simulink model "aerosonde_dynamics_with_autopilot"  (R2021b)
settings: Solver=ode3  StartTime=0.0  StopTime=250  FixedStep=dt  RelTol=1e-6  EnableMultiTasking=on
InitFcn:
  | aerosonde_initialize
  | fault_configurations
  | init_sensor_model
StopFcn:
  | aerosende_grafik;
values from neighbouring files (symbols this model uses):
  aerosonde = AircraftSimData    [aerosonde_data.m]    (also in aerosonde_initialize.m = aerosonde_data)
  aoa_sensor_measurement_limit_rad = deg2rad(30)    [init_sensor_model.m]
  aoa_sensor_noise_power = 0.00030462    [init_sensor_model.m]
  bias_fault_active = TRUE    (= 1)    [fault_configurations.m]
  bias_fault_time = 150    [fault_configurations.m]
  bias_rad = deg2rad(3)    [fault_configurations.m]
  drift_fault_active = FALSE    (= 0)    [fault_configurations.m]
  drift_limit_rad = deg2rad(20)    [fault_configurations.m]
  drift_ratio_rad_s = deg2rad(0.2)    [fault_configurations.m]
  dt = 1/50    (= 0.02)    [aerosonde_initialize.m]
  F = [0 1 0 ... (first row only)    [aerosonde_initialize.m]
  flightconfig = flightconfig_data    [aerosonde_initialize.m]    (also in flightconfig_data.m = siminitialdetails)
  stuck_fault_active = FALSE    (= 0)    [fault_configurations.m]
  x_init = [510.0; -flightconfig.We_VL  ; 0.0]    [aerosonde_initialize.m]
undefined symbols (not defined in the file or in its folder): magnitude, MIL
libraries: simulink_extras x24, simulink x6, aerolibasang x3, aerolibwind2 x3, aerolibbdyn x2, aerolibadyn x1, aerolibtransform2 x1, shareddyn x1, aerolibobsolete x1, sharedutil x1, aerolibatmos2 x1
(part 2 of 2)

== system aerosonde_dynamics_with_autopilot/ UAV Dynamics/Total Moment ==
  note: Sum forces and moments
  note: Total moments at CG location
  Faero : Inport  PortDimensions=3
  Maero : Inport  Port=2  PortDimensions=3
  Fprop : Inport  Port=3  PortDimensions=3
  Mprop : Inport  Port=4  PortDimensions=3
  CGpos : Inport  Port=5  PortDimensions=3
  Moments about CG due to Propulsion Forces : aerolibbdyn/Moments about CG  due to Forces
      settings: SourceProductBaseCode=AE
  Sum1 : Sum  Inputs=+++  InputSameDT=on  SaturateOnIntegerOverflow=on  OutDataTypeStr=Inherit: Same as first input
  Total forces (excluding g) : Sum  InputSameDT=on  SaturateOnIntegerOverflow=on  OutDataTypeStr=Inherit: Same as first input
  r_prop : Constant  Value=aerosonde.rHub  OutDataTypeStr=double
  Fcg : Outport
  Mcg : Outport  Port=2
  wires:
  Maero/1 -> Sum1/2
  Moments about CG due to Propulsion Forces/1 -> Sum1/1
  Total forces (excluding g)/1 -> Fcg/1
  Faero/1 -> Total forces (excluding g)/1
  Fprop/1 -> Total forces (excluding g)/2, Moments about CG due to Propulsion Forces/1
  Mprop/1 -> Sum1/3
  Sum1/1 -> Mcg/1
  r_prop/1 -> Moments about CG due to Propulsion Forces/3
  CGpos/1 -> Moments about CG due to Propulsion Forces/2

== system aerosonde_dynamics_with_autopilot/AoA Sensor Model/Enabled Subsystem ==
  alpha_fault_free : Inport
  Enable : EnablePort
  Add : Sum
  Clock : Clock
  Constant : Constant  Value=bias_fault_time
  Constant1 : Constant  Value=bias_rad
  GreaterThan : RelationalOperator  Operator=>  OutDataTypeStr=boolean  RndMeth=Simplest
  Product : Product
  Transfer Fcn : TransferFcn  Denominator=[0.1 1]
  alpha_biased_rad : Outport
  wires:
  Clock/1 -> GreaterThan/1
  Constant/1 -> GreaterThan/2
  GreaterThan/1 -> Product/1
  Constant1/1 -> Product/2
  Product/1 -> Transfer Fcn/1
  alpha_fault_free/1 -> Add/1
  Transfer Fcn/1 -> Add/2
  Add/1 -> alpha_biased_rad/1

== system aerosonde_dynamics_with_autopilot/AoA Sensor Model/Enabled Subsystem1 ==
  alpha_fault_free : Inport
  Enable : EnablePort
  Add : Sum
  Clock : Clock
  Constant : Constant  Value=bias_fault_time
  Constant1 : Constant  Value=drift_ratio_rad_s
  GreaterThan : RelationalOperator  Operator=>  OutDataTypeStr=boolean  RndMeth=Simplest
  Integrator : Integrator  LimitOutput=on  UpperSaturationLimit=drift_limit_rad  LowerSaturationLimit=-drift_limit_rad
  Product : Product
  alpha_drifted_rad : Outport
  wires:
  Add/1 -> alpha_drifted_rad/1
  Integrator/1 -> Add/2
  alpha_fault_free/1 -> Add/1
  Product/1 -> Integrator/1
  Constant1/1 -> Product/2
  GreaterThan/1 -> Product/1
  Constant/1 -> GreaterThan/2
  Clock/1 -> GreaterThan/1

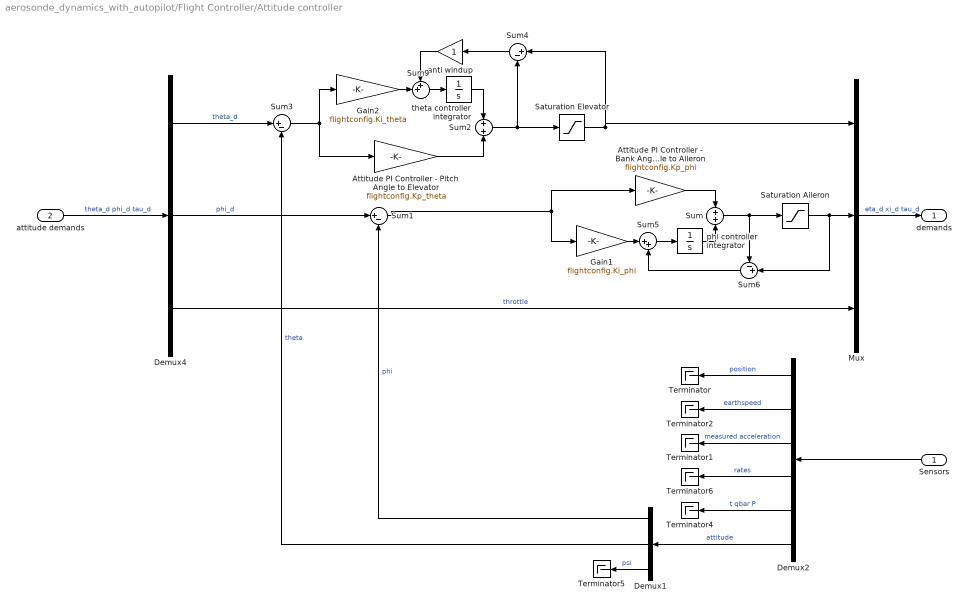
== system aerosonde_dynamics_with_autopilot/Flight Controller/Attitude controller ==
  Sensors : Inport
  attitude demands : Inport  Port=2
  Attitude PI Controller - Bank Angle to Aileron : Gain  Gain=flightconfig.Kp_phi
  Attitude PI Controller - Pitch Angle to Elevator : Gain  Gain=flightconfig.Kp_theta
  Demux1 : Demux  Outputs=3
      settings: DisplayOption=none
  Demux2 : Demux  Outputs=[3 3 3 3 3 3]
  Demux4 : Demux  Outputs=3
      settings: DisplayOption=none
  Gain1 : Gain  Gain=flightconfig.Ki_phi
  Gain2 : Gain  Gain=flightconfig.Ki_theta
  Mux : Mux  Inputs=3
  Saturation Aileron : Saturate  UpperLimit=20*pi/180  LowerLimit=-20*pi/180  ZeroCross=off
  Saturation Elevator : Saturate  UpperLimit=20*pi/180  LowerLimit=-20*pi/180  ZeroCross=off
  Sum : Sum  Inputs=+|+
  Sum1 : Sum  Inputs=|+-
  Sum2 : Sum  Inputs=+|+
  Sum3 : Sum  Inputs=|+-
  Sum4 : Sum  Inputs=|+-
  Sum5 : Sum  Inputs=|++
  Sum6 : Sum  Inputs=-+|
  Sum9 : Sum  Inputs=++|
  Terminator{,1..2,4..6} (6 alike) : Terminator
  anti windup : Gain
  phi controller integrator : Integrator  InitialCondition=flightconfig.xi_trim
  theta controller integrator : Integrator  InitialCondition=flightconfig.eta_trim + flightconfig.Ktheta_eta*flightconfig.theta_trim + flightconfig.Kq_eta*flightconfig.q_trim
  demands : Outport
  wires:
  Sum1/1 -> Attitude PI Controller - Bank Angle to Aileron/1, Gain1/1
  Demux4/2 -> Sum1/1  "phi_d"
  Sum3/1 -> Gain2/1, Attitude PI Controller - Pitch Angle to Elevator/1
  theta controller integrator/1 -> Sum2/1
  Attitude PI Controller - Pitch Angle to Elevator/1 -> Sum2/2
  Gain2/1 -> Sum9/2
  Sum9/1 -> theta controller integrator/1
  Sum2/1 -> Saturation Elevator/1, Sum4/2
  Saturation Elevator/1 -> Sum4/1, Mux/1
  Sum4/1 -> anti windup/1
  anti windup/1 -> Sum9/1
  phi controller integrator/1 -> Sum/2
  Sum/1 -> Saturation Aileron/1, Sum6/1
  Demux4/3 -> Mux/3  "throttle"
  attitude demands/1 -> Demux4/1  "theta_d phi_d tau_d"
  Mux/1 -> demands/1  "eta_d xi_d tau_d"
  Demux4/1 -> Sum3/1  "theta_d"
  Attitude PI Controller - Bank Angle to Aileron/1 -> Sum/1
  Demux2/2 -> Terminator2/1  "earthspeed"
  Demux2/3 -> Terminator1/1  "measured acceleration"
  Sensors/1 -> Demux2/1
  Demux2/5 -> Terminator4/1  "t qbar P"
  Demux2/1 -> Terminator/1  "position"
  Demux2/6 -> Demux1/1  "attitude"
  Demux1/1 -> Sum1/2  "phi"
  Demux1/2 -> Sum3/2  "theta"
  Demux1/3 -> Terminator5/1  "psi"
  Demux2/4 -> Terminator6/1  "rates"
  Saturation Aileron/1 -> Mux/2, Sum6/2
  Gain1/1 -> Sum5/1
  Sum5/1 -> phi controller integrator/1
  Sum6/1 -> Sum5/2

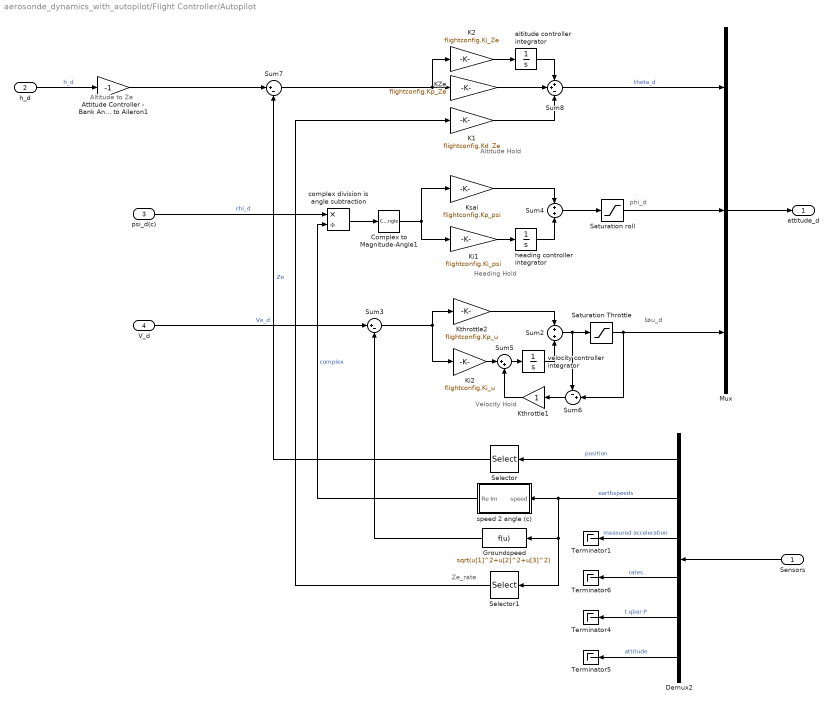
== system aerosonde_dynamics_with_autopilot/Flight Controller/Autopilot ==
  note: Heading Hold
  note: Altitude to Ze
  note: Velocity Hold
  note: Altitude Hold
  note: phi_d
  note: tau_d
  note: Ze_rate
  Sensors : Inport
  h_d : Inport  Port=2
  psi_d(c) : Inport  Port=3
  V_d : Inport  Port=4
  Attitude Controller - Bank Angle to Aileron1 : Gain  Gain=-1
  Complex to Magnitude-Angle1 : ComplexToMagnitudeAngle  Output=Angle
  Demux2 : Demux  Outputs=[3 3 3 3 3 3]
  Groundspeed : Fcn  Expr=sqrt(u[1]^2+u[2]^2+u[3]^2)
  K1 : Gain  Gain=flightconfig.Kd_Ze
  K2 : Gain  Gain=flightconfig.Ki_Ze
  KZe : Gain  Gain=flightconfig.Kp_Ze
  Ki1 : Gain  Gain=flightconfig.Ki_psi
  Ki2 : Gain  Gain=flightconfig.Ki_u
  Ksai : Gain  Gain=flightconfig.Kp_psi
  Kthrottle1 : Gain
  Kthrottle2 : Gain  Gain=flightconfig.Kp_u
  Mux : Mux  Inputs=3
  Saturation Throttle : Saturate  UpperLimit=1  LowerLimit=0  ZeroCross=off
  Saturation roll : Saturate  UpperLimit=1.1  LowerLimit=-1.1  ZeroCross=off
  Selector : Selector  InputPortWidth=3  IndexOptions=Index vector (dialog)  Indices=3  OutputSizes=1
  Selector1 : Selector  InputPortWidth=3  IndexOptions=Index vector (dialog)  Indices=3  OutputSizes=1
  Sum2 : Sum
  Sum3 : Sum  Inputs=|+-
  Sum4 : Sum
  Sum5 : Sum  Inputs=|++
  Sum6 : Sum  Inputs=-+|
  Sum7 : Sum  Inputs=|+-
  Sum8 : Sum  Inputs=++-
  Terminator{1,4..6} (4 alike) : Terminator
  altitude controller integrator : Integrator  InitialCondition=flightconfig.theta_trim  LimitOutput=on  UpperSaturationLimit=.3  LowerSaturationLimit=-.3
  complex division is angle subtraction : Product  Inputs=*/
  heading controller integrator : Integrator  InitialCondition=flightconfig.chi_trim  LimitOutput=on  UpperSaturationLimit=1.2  LowerSaturationLimit=-1.2
  speed 2 angle (c) : Subsystem
  velocity controller integrator : Integrator  InitialCondition=flightconfig.tau_trim
  attitude_d : Outport
  wires:
  Ksai/1 -> Sum4/1
  Sum7/1 -> KZe/1, K2/1
  KZe/1 -> Sum8/2
  K2/1 -> altitude controller integrator/1
  altitude controller integrator/1 -> Sum8/1
  K1/1 -> Sum8/3
  Attitude Controller - Bank Angle to Aileron1/1 -> Sum7/1
  Kthrottle2/1 -> Sum2/1
  Sum2/1 -> Saturation Throttle/1, Sum6/1
  Sum3/1 -> Kthrottle2/1, Ki2/1
  Saturation Throttle/1 -> Sum6/2, Mux/3
  Ki2/1 -> Sum5/1
  Sum5/1 -> velocity controller integrator/1
  velocity controller integrator/1 -> Sum2/2
  Sum6/1 -> Kthrottle1/1
  Kthrottle1/1 -> Sum5/2
  Ki1/1 -> heading controller integrator/1
  h_d/1 -> Attitude Controller - Bank Angle to Aileron1/1  "h_d"
  V_d/1 -> Sum3/1  "Ve_d"
  Sum8/1 -> Mux/1  "theta_d"
  Sum4/1 -> Saturation roll/1
  Demux2/2 -> Groundspeed/1, Selector1/1, speed 2 angle (c)/1(speed)  "earthspeeds"
  Demux2/3 -> Terminator1/1  "measured acceleration"
  Sensors/1 -> Demux2/1
  Demux2/5 -> Terminator4/1  "t qbar P"
  Demux2/1 -> Selector/1  "position"
  Demux2/4 -> Terminator6/1  "rates"
  Demux2/6 -> Terminator5/1  "attitude"
  Groundspeed/1 -> Sum3/2
  heading controller integrator/1 -> Sum4/2
  Selector1/1 -> K1/1
  Mux/1 -> attitude_d/1
  psi_d(c)/1 -> complex division is angle subtraction/1  "chi_d"
  Saturation roll/1 -> Mux/2
  speed 2 angle (c)/1(Re Im) -> complex division is angle subtraction/2  "complex"
  complex division is angle subtraction/1 -> Complex to Magnitude-Angle1/1
  Complex to Magnitude-Angle1/1 -> Ksai/1, Ki1/1
  Selector/1 -> Sum7/2  "Ze"

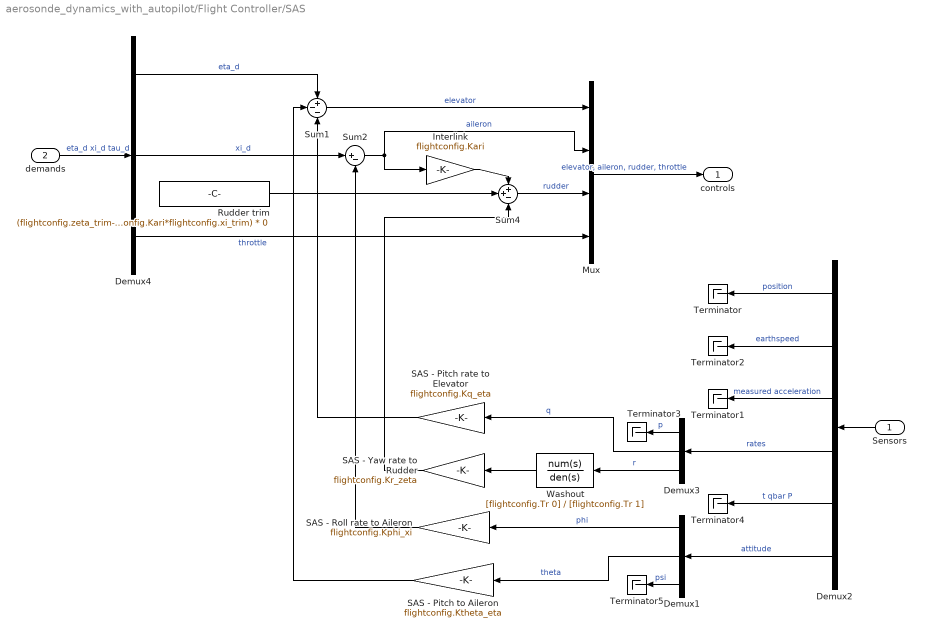
== system aerosonde_dynamics_with_autopilot/Flight Controller/SAS ==
  Sensors : Inport
  demands : Inport  Port=2
  Demux1 : Demux  Outputs=3
      settings: DisplayOption=none
  Demux2 : Demux  Outputs=[3 3 3 3 3 3]
  Demux3 : Demux  Outputs=3
      settings: DisplayOption=none
  Demux4 : Demux  Outputs=3
      settings: DisplayOption=none
  Interlink : Gain  Gain=flightconfig.Kari
  Mux : Mux
  Rudder trim : Constant  Value=(flightconfig.zeta_trim-flightconfig.Kari*flightconfig.xi_trim) * 0
  SAS - Pitch rate to Elevator : Gain  Gain=flightconfig.Kq_eta
  SAS - Pitch to Aileron : Gain  Gain=flightconfig.Ktheta_eta
  SAS - Roll rate to Aileron : Gain  Gain=flightconfig.Kphi_xi
  SAS - Yaw rate to Rudder : Gain  Gain=flightconfig.Kr_zeta
  Sum1 : Sum  Inputs=+--
  Sum2 : Sum  Inputs=|+-
  Sum4 : Sum  Inputs=++-
  Terminator{,1..5} (6 alike) : Terminator
  Washout : TransferFcn  Numerator=[flightconfig.Tr 0]  Denominator=[flightconfig.Tr 1]
  controls : Outport
  wires:
  Washout/1 -> SAS - Yaw rate to Rudder/1
  Demux3/3 -> Washout/1  "r"
  Demux2/2 -> Terminator2/1  "earthspeed"
  Demux2/3 -> Terminator1/1  "measured acceleration"
  Sensors/1 -> Demux2/1
  Demux2/4 -> Demux3/1  "rates"
  Demux2/5 -> Terminator4/1  "t qbar P"
  Demux3/2 -> SAS - Pitch rate to Elevator/1  "q"
  Demux2/1 -> Terminator/1  "position"
  Demux2/6 -> Demux1/1  "attitude"
  Demux3/1 -> Terminator3/1  "p"
  Demux4/3 -> Mux/4  "throttle"
  Sum4/1 -> Mux/3  "rudder"
  Sum1/1 -> Mux/1  "elevator"
  Demux4/1 -> Sum1/1  "eta_d"
  Demux4/2 -> Sum2/1  "xi_d"
  Sum2/1 -> Interlink/1, Mux/2  "aileron"
  Rudder trim/1 -> Sum4/2
  Interlink/1 -> Sum4/1
  Demux1/1 -> SAS - Roll rate to Aileron/1  "phi"
  Demux1/2 -> SAS - Pitch to Aileron/1  "theta"
  SAS - Pitch to Aileron/1 -> Sum1/2
  Demux1/3 -> Terminator5/1  "psi"
  SAS - Yaw rate to Rudder/1 -> Sum4/3
  SAS - Roll rate to Aileron/1 -> Sum2/2
  SAS - Pitch rate to Elevator/1 -> Sum1/3
  Mux/1 -> controls/1  "elevator, aileron, rudder, throttle"
  demands/1 -> Demux4/1  "eta_d xi_d tau_d"

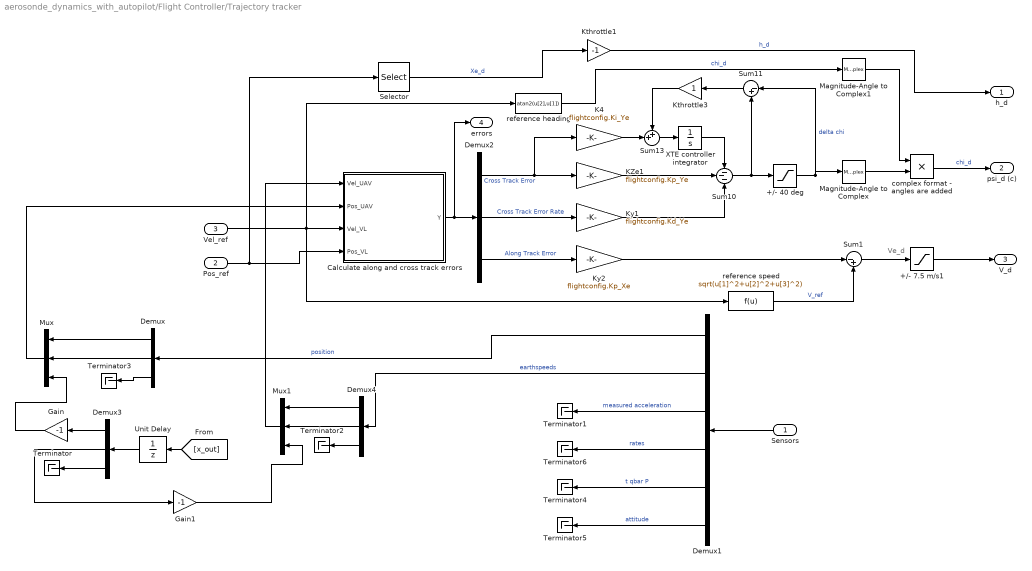
== system aerosonde_dynamics_with_autopilot/Flight Controller/Trajectory tracker ==
  note: Ve_d
  Sensors : Inport  PortDimensions=18
  Pos_ref : Inport  Port=2
  Vel_ref : Inport  Port=3
  +/- 40 deg : Saturate  UpperLimit=+40.0*pi/180  LowerLimit=-40*pi/180  ZeroCross=off
  +/- 7.5 m/s1 : Saturate  UpperLimit=90  LowerLimit=18  ZeroCross=off
  Calculate along and cross track errors : MATLAB Function  TreatAsAtomicUnit=on
  Demux{,2..4} (4 alike) : Demux  Outputs=3
  Demux1 : Demux  Outputs=[3 3 3 3 3 3]
  Gain : Gain  Gain=-1
  Gain1 : Gain  Gain=-1
  K4 : Gain  Gain=flightconfig.Ki_Ye
  KZe1 : Gain  Gain=flightconfig.Kp_Ye
  Kthrottle1 : Gain  Gain=-1
  Kthrottle3 : Gain
  Ky1 : Gain  Gain=flightconfig.Kd_Ye
  Ky2 : Gain  Gain=flightconfig.Kp_Xe
  Magnitude-Angle to Complex : MagnitudeAngleToComplex  Input=Angle  ConstantPart=1
  Magnitude-Angle to Complex1 : MagnitudeAngleToComplex  Input=Angle  ConstantPart=1
  Mux : Mux  Inputs=3
  Mux1 : Mux  Inputs=3
  Selector : Selector  InputPortWidth=3  IndexOptions=Index vector (dialog)  Indices=3  OutputSizes=1
  Sum1 : Sum  Inputs=|-+
  Sum10 : Sum  Inputs=---
  Sum11 : Sum  Inputs=|-+
  Sum13 : Sum  Inputs=++|
  Terminator{,1..6} (7 alike) : Terminator
  Unit Delay : UnitDelay  InitialCondition=x_init  SampleTime=-1  HasFrameUpgradeWarning=on
  XTE controller integrator : Integrator
  complex format - angles are added : Product  RndMeth=Zero
  reference heading : Fcn  Expr=atan2(u[2],u[1])
  reference speed : Fcn  Expr=sqrt(u[1]^2+u[2]^2+u[3]^2)
  h_d : Outport
  psi_d (c) : Outport  Port=2
  V_d : Outport  Port=3
  errors : Outport  Port=4
  wires:
  KZe1/1 -> Sum10/2
  K4/1 -> Sum13/2
  Sum13/1 -> XTE controller integrator/1
  XTE controller integrator/1 -> Sum10/1
  Sum10/1 -> +/- 40 deg/1, Sum11/2
  Sum11/1 -> Kthrottle3/1
  Kthrottle3/1 -> Sum13/1
  Ky1/1 -> Sum10/3
  Demux2/1 -> KZe1/1, K4/1  "Cross Track Error"
  Calculate along and cross track errors/1(Y) -> Demux2/1, errors/1
  Ky2/1 -> Sum1/1
  Pos_ref/1 -> Calculate along and cross track errors/4(Pos_VL), Selector/1
  Vel_ref/1 -> Calculate along and cross track errors/3(Vel_VL), reference speed/1, reference heading/1
  Demux2/3 -> Ky2/1  "Along Track Error"
  Demux2/2 -> Ky1/1  "Cross Track Error Rate"
  Demux1/2 -> Demux4/1  "earthspeeds"
  Demux1/3 -> Terminator1/1  "measured acceleration"
  Sensors/1 -> Demux1/1
  Demux1/5 -> Terminator4/1  "t qbar P"
  Demux1/1 -> Demux/1  "position"
  Demux1/4 -> Terminator6/1  "rates"
  Demux1/6 -> Terminator5/1  "attitude"
  Selector/1 -> Kthrottle1/1  "Xe_d"
  Kthrottle1/1 -> h_d/1  "h_d"
  Sum1/1 -> +/- 7.5 m/s1/1
  reference speed/1 -> Sum1/2  "V_ref"
  +/- 7.5 m/s1/1 -> V_d/1
  complex format - angles are added/1 -> psi_d (c)/1  "chi_d"
  +/- 40 deg/1 -> Sum11/1, Magnitude-Angle to Complex/1  "delta chi"
  reference heading/1 -> Magnitude-Angle to Complex1/1  "chi_d"
  Magnitude-Angle to Complex/1 -> complex format - angles are added/2
  Magnitude-Angle to Complex1/1 -> complex format - angles are added/1
  Demux/1 -> Mux/1
  Demux/2 -> Mux/2
  [x_out] -> Unit Delay/1
  Gain/1 -> Mux/3
  Mux/1 -> Calculate along and cross track errors/2(Pos_UAV)
  Demux3/1 -> Gain/1
  Demux3/2 -> Gain1/1
  Demux3/3 -> Terminator/1
  Demux4/1 -> Mux1/1
  Demux4/2 -> Mux1/2
  Gain1/1 -> Mux1/3
  Demux4/3 -> Terminator2/1
  Demux/3 -> Terminator3/1
  Mux1/1 -> Calculate along and cross track errors/1(Vel_UAV)
  Unit Delay/1 -> Demux3/1

== system aerosonde_dynamics_with_autopilot/ UAV Dynamics/Aerodynamics/Force Coefficients ==
  note: Force coefficients
  VBetaAlpha : Inport  PortDimensions=[3 1]
  Control : Inport  Port=2  PortDimensions=[4 1]
  AlphaDot : Inport  Port=3
  AngularRates : Inport  Port=4  PortDimensions=[3 1]
  Mach : Inport  Port=5  PortDimensions=1
  2c : Gain  Gain=2  SaturateOnIntegerOverflow=on  OutDataTypeStr=Inherit: Same as input  ParamDataTypeStr=Inherit: Same as input
  ChSign : Gain  Gain=-1  SaturateOnIntegerOverflow=on  OutDataTypeStr=Inherit: Same as input  ParamDataTypeStr=Inherit: Same as input
  ChSign1 : Gain  Gain=-1  SaturateOnIntegerOverflow=on  OutDataTypeStr=Inherit: Same as input  ParamDataTypeStr=Inherit: Same as input
  DCM' : Math  Operator=transpose  SignedPower=on  SaturateOnIntegerOverflow=on
  Demux2 : Demux  Outputs=3
      settings: DisplayOption=none
  Direction Cosine Matrix Body to Wind : aerolibtransform2/Direction Cosine Matrix Body to Wind
      settings: SourceProductBaseCode=AE
  Drag Coefficients : Subsystem
  Lift Coefficients : Subsystem
  Mux : Mux  Inputs=3
  Mux1 : Mux  Inputs=2
  Side Force Coefficients : Subsystem
  transform to body axes : Product  Inputs=**  Multiplication=Matrix(*)  InputSameDT=on  SaturateOnIntegerOverflow=on  OutDataTypeStr=Inherit: Same as first input
  "[-CD, CY, -CL]" : Outport
  wires:
  Mux1/1 -> Direction Cosine Matrix Body to Wind/1
  DCM'/1 -> transform to body axes/1
  Mux/1 -> transform to body axes/2
  Direction Cosine Matrix Body to Wind/1 -> DCM'/1
  transform to body axes/1 -> "[-CD, CY, -CL]"/1
  Demux2/2 -> Mux1/2, Side Force Coefficients/1(beta)
  Demux2/1 -> 2c/1
  VBetaAlpha/1 -> Demux2/1
  ChSign1/1 -> Mux/3
  ChSign/1 -> Mux/1
  Side Force Coefficients/1(CY) -> Mux/2
  Drag Coefficients/1(CD) -> ChSign/1
  Lift Coefficients/1(CL) -> Drag Coefficients/3(CL), ChSign1/1
  Mach/1 -> Drag Coefficients/2(Mach), Lift Coefficients/6(Mach)
  AngularRates/1 -> Side Force Coefficients/3(angular rates), Lift Coefficients/4(pqr)
  AlphaDot/1 -> Lift Coefficients/3(alphadot)
  Control/1 -> Side Force Coefficients/2(control), Lift Coefficients/2(control), Drag Coefficients/1(control)
  Demux2/3 -> Lift Coefficients/1(alpha), Mux1/1
  2c/1 -> Side Force Coefficients/4(2V_a), Lift Coefficients/5(2V_a)

== system aerosonde_dynamics_with_autopilot/ UAV Dynamics/Aerodynamics/Moment Coefficients ==
  note: Moment coefficients
  VBetaAlpha : Inport  PortDimensions=[3 1]
  Control : Inport  Port=2  PortDimensions=[4 1]
  AlphaDot : Inport  Port=3
  AngularRates : Inport  Port=4  PortDimensions=[3 1]
  Mach : Inport  Port=5  PortDimensions=1
  2c : Gain  Gain=2  SaturateOnIntegerOverflow=on  OutDataTypeStr=Inherit: Same as input  ParamDataTypeStr=Inherit: Same as input
  Demux1 : Demux  Outputs=3
      settings: DisplayOption=none
  Mux : Mux  Inputs=3
  Pitch Moment Coefficients : Subsystem
  Roll Moment Coefficients : Subsystem
  Yaw Moment Coefficients : Subsystem
  "[-Cl, Cm, -Cn]" : Outport
  wires:
  Demux1/2 -> Yaw Moment Coefficients/1(beta), Roll Moment Coefficients/1(beta)
  Demux1/3 -> Pitch Moment Coefficients/1(alpha)
  Mach/1 -> Pitch Moment Coefficients/6(Mach)
  Yaw Moment Coefficients/1(Cn) -> Mux/3
  VBetaAlpha/1 -> Demux1/1
  2c/1 -> Pitch Moment Coefficients/5(2V_a), Yaw Moment Coefficients/4(2V_a), Roll Moment Coefficients/4(2V)
  Demux1/1 -> 2c/1
  Control/1 -> Yaw Moment Coefficients/2(control), Pitch Moment Coefficients/2(control), Roll Moment Coefficients/2(control)
  AlphaDot/1 -> Pitch Moment Coefficients/3(alphadot)
  AngularRates/1 -> Roll Moment Coefficients/3(angular rates), Yaw Moment Coefficients/3(angular rates), Pitch Moment Coefficients/4(pqr)
  Mux/1 -> "[-Cl, Cm, -Cn]"/1
  Pitch Moment Coefficients/1(Cm) -> Mux/2
  Roll Moment Coefficients/1(Cl) -> Mux/1

== system aerosonde_dynamics_with_autopilot/ UAV Dynamics/Aerodynamics/Wind-axes Velocities ==
  VelB : Inport
  WindB : Inport  Port=2
  a : Inport  Port=3
  rho : Inport  Port=4
  VelBdot : Inport  Port=5
  Calculate alphadot : Subsystem
  Derivative : Derivative
  Dynamic Pressure : aerolibasang/Dynamic Pressure
  "Incidence, Sideslip, & Airspeed" : aerolibasang/Incidence, Sideslip, & Airspeed
  Mach Number : aerolibasang/Mach Number
      settings: SourceProductBaseCode=AE
  Mux1 : Mux  Inputs=3
  Sum1 : Sum  Inputs=|+-  InputSameDT=on  SaturateOnIntegerOverflow=on  OutDataTypeStr=Inherit: Same as first input
  Sum2 : Sum  Inputs=-+|  InputSameDT=on  SaturateOnIntegerOverflow=on  OutDataTypeStr=Inherit: Same as first input
  VBetaAlpha : Outport
  Mach : Outport  Port=2
  qbar (pdyn) : Outport  Port=3
  alphadot : Outport  Port=4
  wires:
  Derivative/1 -> Sum2/1
  Sum2/1 -> Calculate alphadot/1("[Udot Vdot Wdot]")
  VelBdot/1 -> Sum2/2
  Calculate alphadot/1(alphadot) -> alphadot/1
  "Incidence, Sideslip, & Airspeed"/2 -> Mux1/2
  "Incidence, Sideslip, & Airspeed"/1 -> Mux1/3
  Dynamic Pressure/1 -> qbar (pdyn)/1
  rho/1 -> Dynamic Pressure/2
  a/1 -> Mach Number/2
  Mach Number/1 -> Mach/1
  WindB/1 -> Derivative/1, Sum1/2
  VelB/1 -> Sum1/1
  Mux1/1 -> VBetaAlpha/1
  "Incidence, Sideslip, & Airspeed"/3 -> Mux1/1
  Sum1/1 -> Calculate alphadot/2("[U V W]"), Dynamic Pressure/1, Mach Number/1, "Incidence, Sideslip, & Airspeed"/1

== system aerosonde_dynamics_with_autopilot/ UAV Dynamics/Propulsion System/Fixed-pitch Propeller ==
  note: Fixed-pitch
      | Propeller
  Airspeed : Inport  OutDataTypeStr=double  PortDimensions=1
  rho : Inport  Port=2  OutDataTypeStr=double  PortDimensions=1
  Omega : Inport  Port=3  OutDataTypeStr=double  PortDimensions=1
  4 R^4 / pi^2 : Gain  Gain=4*Rprop^4/pi^2  SaturateOnIntegerOverflow=on  OutDataTypeStr=Inherit: Same as input  ParamDataTypeStr=Inherit: Same as input
  4 R^5/ pi^3 : Gain  Gain=-4*Rprop^5/pi^3  SaturateOnIntegerOverflow=on  OutDataTypeStr=Inherit: Same as input  ParamDataTypeStr=Inherit: Same as input
  Coeff of Power : Lookup_n-D  NumberOfTableDimensions=1  BreakpointsForDimension1=J  Table=CP  InternalRulePriority=Speed  SaturateOnIntegerOverflow=on  InputSameDT=on
  Coefficient of Thrust : Lookup_n-D  NumberOfTableDimensions=1  BreakpointsForDimension1=J  Table=CT  InternalRulePriority=Speed  SaturateOnIntegerOverflow=on  InputSameDT=on
  Omega^2 : Math  Operator=square  SignedPower=on  SaturateOnIntegerOverflow=on
  Va/Omega : Product  Inputs=*/  InputSameDT=on  SaturateOnIntegerOverflow=on  OutDataTypeStr=Inherit: Same as first input
  pi/R : Gain  Gain=pi/Rprop  SaturateOnIntegerOverflow=on  OutDataTypeStr=Inherit: Same as input  ParamDataTypeStr=Inherit: Same as input
  "rho Omega^2 " : Product  InputSameDT=on  SaturateOnIntegerOverflow=on  OutDataTypeStr=Inherit: Same as first input
  rho Omega^2 C_P : Product  InputSameDT=on  SaturateOnIntegerOverflow=on  OutDataTypeStr=Inherit: Same as first input
  rho Omega^2 C_T : Product  InputSameDT=on  SaturateOnIntegerOverflow=on  OutDataTypeStr=Inherit: Same as first input
  Fprop : Outport
  Mprop : Outport  Port=2
  wires:
  "rho Omega^2 "/1 -> rho Omega^2 C_P/2, rho Omega^2 C_T/2
  Omega^2/1 -> "rho Omega^2 "/1
  rho/1 -> "rho Omega^2 "/2
  4 R^5/ pi^3/1 -> Mprop/1  "torque"
  4 R^4 / pi^2/1 -> Fprop/1  "thrust"
  Airspeed/1 -> Va/Omega/1
  pi/R/1 -> Coeff of Power/1, Coefficient of Thrust/1  "advance ratio"
  rho Omega^2 C_P/1 -> 4 R^5/ pi^3/1
  rho Omega^2 C_T/1 -> 4 R^4 / pi^2/1
  Coefficient of Thrust/1 -> rho Omega^2 C_T/1
  Va/Omega/1 -> pi/R/1
  Omega/1 -> Va/Omega/2, Omega^2/1
  Coeff of Power/1 -> rho Omega^2 C_P/1

== system aerosonde_dynamics_with_autopilot/ UAV Dynamics/Propulsion System/Piston Engine ==
  note: Compute MAP from
      | throttle area fraction
  note: Engine parameter
      | look-up tables
  Thr : Inport  OutDataTypeStr=double  PortDimensions=1
  Mix : Inport  Port=2  OutDataTypeStr=double  PortDimensions=1
  Omega : Inport  Port=3  OutDataTypeStr=double  PortDimensions=1
  P_atm : Inport  Port=4  OutDataTypeStr=double  PortDimensions=1
  T : Inport  Port=5  OutDataTypeStr=double  PortDimensions=1
  Altitude correction for  Power : Subsystem
  Engine torque : Product  Inputs=*/  InputSameDT=on  SaturateOnIntegerOverflow=on  OutDataTypeStr=Inherit: Same as first input
  Fuel flow LUT : Lookup_n-D  BreakpointsForDimension1=RPM  BreakpointsForDimension2=MAP  BeginIndexSearchUsingPreviousIndexResult=on  Table=fflow  InputSameDT=on
      settings: InputPortMap=u0,u1
  Get air flow : Product  InputSameDT=on  SaturateOnIntegerOverflow=on  OutDataTypeStr=Inherit: Same as first input
  Intake : Subsystem
  Power LUT : Lookup_n-D  BreakpointsForDimension1=RPM  BreakpointsForDimension2=MAP  BeginIndexSearchUsingPreviousIndexResult=on  Table=Power  InputSameDT=on
      settings: InputPortMap=u0,u1
  Power at altitude : Product  InputSameDT=on  SaturateOnIntegerOverflow=on  OutDataTypeStr=Inherit: Same as first input
  g/hr 2 kg/s : Gain  Gain=1/1000/3600  SaturateOnIntegerOverflow=on  OutDataTypeStr=Inherit: Same as input  ParamDataTypeStr=Inherit: Same as input
  rad/s 2 RPM : Gain  Gain=30/pi  SaturateOnIntegerOverflow=on  OutDataTypeStr=Inherit: Same as input  ParamDataTypeStr=Inherit: Same as input
  AirFlow : Outport
  FuelFlow : Outport  Port=2
  Torque : Outport  Port=3
  wires:
  Get air flow/1 -> AirFlow/1
  Mix/1 -> Get air flow/2
  Intake/1(MAP) -> Power LUT/2, Fuel flow LUT/2
  g/hr 2 kg/s/1 -> Get air flow/1, FuelFlow/1
  Omega/1 -> rad/s 2 RPM/1, Engine torque/2
  rad/s 2 RPM/1 -> Fuel flow LUT/1, Power LUT/1
  T/1 -> Altitude correction for  Power/1(T)
  Power LUT/1 -> Power at altitude/1
  Altitude correction for  Power/1(Power correction) -> Power at altitude/2
  Power at altitude/1 -> Engine torque/1
  Engine torque/1 -> Torque/1
  Thr/1 -> Intake/1(Thr)
  P_atm/1 -> Intake/2(P_atm)
  Fuel flow LUT/1 -> g/hr 2 kg/s/1

== system aerosonde_dynamics_with_autopilot/Flight Controller/Autopilot/speed 2 angle (c) ==
  speed : Inport
  Demux : Demux  Outputs=3
  Real-Imag to Complex : RealImagToComplex
  Terminator2 : Terminator
  Re Im : Outport
  wires:
  speed/1 -> Demux/1
  Real-Imag to Complex/1 -> Re Im/1
  Demux/3 -> Terminator2/1
  Demux/2 -> Real-Imag to Complex/2
  Demux/1 -> Real-Imag to Complex/1

== system aerosonde_dynamics_with_autopilot/ UAV Dynamics/Aerodynamics/Force Coefficients/Drag Coefficients ==
  note: Drag coefficient
  control : Inport
  Mach : Inport  Port=2
  CL : Inport  Port=3  PortDimensions=1
  (CL-CL0)^2/(pi e AR) : Gain  Gain=1/aerosonde.pieaR  Multiplication=Matrix(K*u)  SaturateOnIntegerOverflow=on  OutDataTypeStr=Inherit: Same as input  ParamDataTypeStr=Inherit: Same as input
  Abs4 : Abs  SaturateOnIntegerOverflow=on
  CDM : Gain  Gain=aerosonde.pCDM  SaturateOnIntegerOverflow=on  OutDataTypeStr=Inherit: Same as input  ParamDataTypeStr=Inherit: Same as input
  CDdf : Gain  Gain=[aerosonde.CDdf, aerosonde.CDde, aerosonde.CDda, aerosonde.CDdr]  Multiplication=Matrix(K*u)  SaturateOnIntegerOverflow=on  OutDataTypeStr=Inherit: Same as input  ParamDataTypeStr=Inherit: Same as input
  CL min drag : Constant  Value=aerosonde.CLmind
  CL^2 : Math  Operator=square  SignedPower=on  SaturateOnIntegerOverflow=on
  Constant terms : Constant  Value=aerosonde.CD0
  Sum : Sum  Inputs=|+-  InputSameDT=on  SaturateOnIntegerOverflow=on  OutDataTypeStr=Inherit: Same as first input
  Sum1 : Sum  Inputs=++++  InputSameDT=on  SaturateOnIntegerOverflow=on  OutDataTypeStr=Inherit: Same as first input
  CD : Outport
  wires:
  (CL-CL0)^2/(pi e AR)/1 -> Sum1/4
  CL min drag/1 -> Sum/2
  CL/1 -> Sum/1
  Sum/1 -> CL^2/1
  CL^2/1 -> (CL-CL0)^2/(pi e AR)/1
  Sum1/1 -> CD/1  "CD"
  Mach/1 -> CDM/1
  control/1 -> Abs4/1
  Abs4/1 -> CDdf/1
  CDM/1 -> Sum1/3
  CDdf/1 -> Sum1/2
  Constant terms/1 -> Sum1/1

== system aerosonde_dynamics_with_autopilot/ UAV Dynamics/Aerodynamics/Force Coefficients/Lift Coefficients ==
  note: Lift Coefficients
  alpha : Inport
  control : Inport  Port=2
  alphadot : Inport  Port=3
  pqr : Inport  Port=4
  2V_a : Inport  Port=5
  Mach : Inport  Port=6
  CL*c/(2V_a) : Product  Inputs=*/  InputSameDT=on  SaturateOnIntegerOverflow=on  OutDataTypeStr=Inherit: Same as first input
  CL0 : Constant  Value=aerosonde.CL0
  CLM : Gain  Gain=aerosonde.CLM  SaturateOnIntegerOverflow=on  OutDataTypeStr=Inherit: Same as input  ParamDataTypeStr=Inherit: Same as input
  CLalpha : Gain  Gain=aerosonde.CLalpha  SaturateOnIntegerOverflow=on  OutDataTypeStr=Inherit: Same as input  ParamDataTypeStr=Inherit: Same as input
  CLalphadot : Gain  Gain=aerosonde.CLalphadot  Multiplication=Matrix(K*u)  SaturateOnIntegerOverflow=on  OutDataTypeStr=Inherit: Same as input  ParamDataTypeStr=Inherit: Same as input
  CLq : Gain  Gain=[0, aerosonde.CLq, 0]  Multiplication=Matrix(K*u)  SaturateOnIntegerOverflow=on  OutDataTypeStr=Inherit: Same as input  ParamDataTypeStr=Inherit: Same as input
  Sum : Sum  InputSameDT=on  SaturateOnIntegerOverflow=on  OutDataTypeStr=Inherit: Same as first input
  Sum2 : Sum  Inputs=+++++  InputSameDT=on  SaturateOnIntegerOverflow=on  OutDataTypeStr=Inherit: Same as first input
  "[CLdf, CLde, 0, 0]" : Gain  Gain=[aerosonde.CLdf, aerosonde.CLde, 0, 0]  Multiplication=Matrix(K*u)  SaturateOnIntegerOverflow=on  OutDataTypeStr=Inherit: Same as input  ParamDataTypeStr=Inherit: Same as input
  c : Gain  Gain=aerosonde.c  SaturateOnIntegerOverflow=on  OutDataTypeStr=Inherit: Same as input  ParamDataTypeStr=Inherit: Same as input
  CL : Outport
  wires:
  alphadot/1 -> CLalphadot/1
  alpha/1 -> CLalpha/1
  Mach/1 -> CLM/1
  2V_a/1 -> CL*c/(2V_a)/2
  pqr/1 -> CLq/1
  control/1 -> "[CLdf, CLde, 0, 0]"/1
  c/1 -> CL*c/(2V_a)/1
  CL*c/(2V_a)/1 -> Sum2/4
  CLM/1 -> Sum2/5
  Sum2/1 -> CL/1  "CL"
  "[CLdf, CLde, 0, 0]"/1 -> Sum2/3
  CLalpha/1 -> Sum2/2
  CL0/1 -> Sum2/1
  Sum/1 -> c/1
  CLalphadot/1 -> Sum/1
  CLq/1 -> Sum/2

== system aerosonde_dynamics_with_autopilot/ UAV Dynamics/Aerodynamics/Force Coefficients/Side Force Coefficients ==
  note: Side force coefficients
  beta : Inport
  control : Inport  Port=2
  angular rates : Inport  Port=3
  2V_a : Inport  Port=4
  CY*b/(2V_a) : Product  Inputs=*/  InputSameDT=on  SaturateOnIntegerOverflow=on  OutDataTypeStr=Inherit: Same as first input
  CYbeta : Gain  Gain=aerosonde.CYbeta  SaturateOnIntegerOverflow=on  OutDataTypeStr=Inherit: Same as input  ParamDataTypeStr=Inherit: Same as input
  Sum3 : Sum  Inputs=+++  InputSameDT=on  SaturateOnIntegerOverflow=on  OutDataTypeStr=Inherit: Same as first input
  Wing span1 : Gain  Gain=aerosonde.b  SaturateOnIntegerOverflow=on  OutDataTypeStr=Inherit: Same as input  ParamDataTypeStr=Inherit: Same as input
  "[0, 0, CYda, CYdr]" : Gain  Gain=[0, 0, aerosonde.CYda, aerosonde.CYdr]  Multiplication=Matrix(K*u)  SaturateOnIntegerOverflow=on  OutDataTypeStr=Inherit: Same as input  ParamDataTypeStr=Inherit: Same as input
  "[CYp, 0, CYr]" : Gain  Gain=[aerosonde.CYp, 0, aerosonde.CYr]  Multiplication=Matrix(K*u)  SaturateOnIntegerOverflow=on  OutDataTypeStr=Inherit: Same as input  ParamDataTypeStr=Inherit: Same as input
  CY : Outport
  wires:
  beta/1 -> CYbeta/1
  2V_a/1 -> CY*b/(2V_a)/2
  angular rates/1 -> "[CYp, 0, CYr]"/1
  control/1 -> "[0, 0, CYda, CYdr]"/1
  Wing span1/1 -> CY*b/(2V_a)/1
  Sum3/1 -> CY/1  "CY"
  CY*b/(2V_a)/1 -> Sum3/3
  "[0, 0, CYda, CYdr]"/1 -> Sum3/2
  CYbeta/1 -> Sum3/1
  "[CYp, 0, CYr]"/1 -> Wing span1/1

== system aerosonde_dynamics_with_autopilot/ UAV Dynamics/Aerodynamics/Moment Coefficients/Pitch Moment Coefficients ==
  alpha : Inport
  control : Inport  Port=2
  alphadot : Inport  Port=3
  pqr : Inport  Port=4
  2V_a : Inport  Port=5
  Mach : Inport  Port=6
  CMalpha : Gain  Gain=aerosonde.Cmalpha  SaturateOnIntegerOverflow=on  OutDataTypeStr=Inherit: Same as input  ParamDataTypeStr=Inherit: Same as input
  Cm*c/(2V_a) : Product  Inputs=*/  InputSameDT=on  SaturateOnIntegerOverflow=on  OutDataTypeStr=Inherit: Same as first input
  Cm0 : Constant  Value=aerosonde.Cm0
  CmM : Gain  Gain=aerosonde.CmM  SaturateOnIntegerOverflow=on  OutDataTypeStr=Inherit: Same as input  ParamDataTypeStr=Inherit: Same as input
  Cmalphadot : Gain  Gain=aerosonde.Cmalphadot  Multiplication=Matrix(K*u)  SaturateOnIntegerOverflow=on  OutDataTypeStr=Inherit: Same as input  ParamDataTypeStr=Inherit: Same as input
  Cmq : Gain  Gain=[0, aerosonde.Cmq, 0]  Multiplication=Matrix(K*u)  SaturateOnIntegerOverflow=on  OutDataTypeStr=Inherit: Same as input  ParamDataTypeStr=Inherit: Same as input
  Sum : Sum  InputSameDT=on  SaturateOnIntegerOverflow=on  OutDataTypeStr=Inherit: Same as first input
  Sum2 : Sum  Inputs=+++++  InputSameDT=on  SaturateOnIntegerOverflow=on  OutDataTypeStr=Inherit: Same as first input
  "[Cmdf, Cmde, 0, 0]" : Gain  Gain=[aerosonde.Cmdf, aerosonde.Cmde, 0, 0]  Multiplication=Matrix(K*u)  SaturateOnIntegerOverflow=on  OutDataTypeStr=Inherit: Same as input  ParamDataTypeStr=Inherit: Same as input
  c : Gain  Gain=aerosonde.c  SaturateOnIntegerOverflow=on  OutDataTypeStr=Inherit: Same as input  ParamDataTypeStr=Inherit: Same as input
  Cm : Outport
  wires:
  Cmq/1 -> Sum/2
  Cmalphadot/1 -> Sum/1
  Sum/1 -> c/1
  Cm0/1 -> Sum2/1
  CMalpha/1 -> Sum2/2
  "[Cmdf, Cmde, 0, 0]"/1 -> Sum2/3
  Sum2/1 -> Cm/1  "Cm"
  CmM/1 -> Sum2/5
  Cm*c/(2V_a)/1 -> Sum2/4
  c/1 -> Cm*c/(2V_a)/1
  control/1 -> "[Cmdf, Cmde, 0, 0]"/1
  pqr/1 -> Cmq/1
  2V_a/1 -> Cm*c/(2V_a)/2
  Mach/1 -> CmM/1
  alpha/1 -> CMalpha/1
  alphadot/1 -> Cmalphadot/1

== system aerosonde_dynamics_with_autopilot/ UAV Dynamics/Aerodynamics/Moment Coefficients/Roll Moment Coefficients ==
  note: Roll moment coefficient
  beta : Inport
  control : Inport  Port=2
  angular rates : Inport  Port=3
  2V : Inport  Port=4
  CY*b/(2V) : Product  Inputs=*/  InputSameDT=on  SaturateOnIntegerOverflow=on  OutDataTypeStr=Inherit: Same as first input
  Clbeta : Gain  Gain=aerosonde.Clbeta  SaturateOnIntegerOverflow=on  OutDataTypeStr=Inherit: Same as input  ParamDataTypeStr=Inherit: Same as input
  Sum3 : Sum  Inputs=+++  InputSameDT=on  SaturateOnIntegerOverflow=on  OutDataTypeStr=Inherit: Same as first input
  Wing span : Gain  Gain=aerosonde.b  SaturateOnIntegerOverflow=on  OutDataTypeStr=Inherit: Same as input  ParamDataTypeStr=Inherit: Same as input
  "[0, 0, Clda, Cldr]" : Gain  Gain=[0, 0, aerosonde.Clda, aerosonde.Cldr]  Multiplication=Matrix(K*u)  SaturateOnIntegerOverflow=on  OutDataTypeStr=Inherit: Same as input  ParamDataTypeStr=Inherit: Same as input
  "[Clp, 0, Clr]" : Gain  Gain=[aerosonde.Clp, 0, aerosonde.Clr]  Multiplication=Matrix(K*u)  SaturateOnIntegerOverflow=on  OutDataTypeStr=Inherit: Same as input  ParamDataTypeStr=Inherit: Same as input
  Cl : Outport
  wires:
  "[Clp, 0, Clr]"/1 -> Wing span/1
  Clbeta/1 -> Sum3/1
  "[0, 0, Clda, Cldr]"/1 -> Sum3/2
  CY*b/(2V)/1 -> Sum3/3
  Sum3/1 -> Cl/1  "Cl"
  Wing span/1 -> CY*b/(2V)/1
  control/1 -> "[0, 0, Clda, Cldr]"/1
  angular rates/1 -> "[Clp, 0, Clr]"/1
  2V/1 -> CY*b/(2V)/2
  beta/1 -> Clbeta/1

== system aerosonde_dynamics_with_autopilot/ UAV Dynamics/Aerodynamics/Moment Coefficients/Yaw Moment Coefficients ==
  note: Yaw moment coefficient
  beta : Inport
  control : Inport  Port=2
  angular rates : Inport  Port=3
  2V_a : Inport  Port=4
  Cn*b/(2V_a) : Product  Inputs=*/  InputSameDT=on  SaturateOnIntegerOverflow=on  OutDataTypeStr=Inherit: Same as first input
  Cnbeta : Gain  Gain=aerosonde.Cnbeta*3  SaturateOnIntegerOverflow=on  OutDataTypeStr=Inherit: Same as input  ParamDataTypeStr=Inherit: Same as input
  Sum3 : Sum  Inputs=+++  InputSameDT=on  SaturateOnIntegerOverflow=on  OutDataTypeStr=Inherit: Same as first input
  Wing span : Gain  Gain=aerosonde.b  SaturateOnIntegerOverflow=on  OutDataTypeStr=Inherit: Same as input  ParamDataTypeStr=Inherit: Same as input
  "[0, 0, Cnda, Cndr]" : Gain  Gain=[0, 0, aerosonde.Cnda, aerosonde.Cndr]  Multiplication=Matrix(K*u)  SaturateOnIntegerOverflow=on  OutDataTypeStr=Inherit: Same as input  ParamDataTypeStr=Inherit: Same as input
  "[Cnp, 0, Cnr]" : Gain  Gain=[aerosonde.Cnp, 0, aerosonde.Cnr]  Multiplication=Matrix(K*u)  SaturateOnIntegerOverflow=on  OutDataTypeStr=Inherit: Same as input  ParamDataTypeStr=Inherit: Same as input
  Cn : Outport
  wires:
  beta/1 -> Cnbeta/1
  2V_a/1 -> Cn*b/(2V_a)/2
  angular rates/1 -> "[Cnp, 0, Cnr]"/1
  control/1 -> "[0, 0, Cnda, Cndr]"/1
  Wing span/1 -> Cn*b/(2V_a)/1
  Sum3/1 -> Cn/1  "Cn"
  Cn*b/(2V_a)/1 -> Sum3/3
  "[0, 0, Cnda, Cndr]"/1 -> Sum3/2
  Cnbeta/1 -> Sum3/1
  "[Cnp, 0, Cnr]"/1 -> Wing span/1

== system aerosonde_dynamics_with_autopilot/ UAV Dynamics/Aerodynamics/Wind-axes Velocities/Calculate alphadot ==
  note: Calculate alphadot
  note: W
  "[Udot Vdot Wdot]" : Inport
  "[U V W]" : Inport  Port=2
  Demux : Demux  Outputs=3
  Demux1 : Demux  Outputs=3
  Math Function : Math  Operator=square  SignedPower=on  SaturateOnIntegerOverflow=on
  Math Function1 : Math  Operator=square  SignedPower=on  SaturateOnIntegerOverflow=on
  Product : Product  RndMeth=Zero
  Product1 : Product  RndMeth=Zero
  Product2 : Product  Inputs=*/  RndMeth=Zero
  Sum : Sum  Inputs=-|+
  Sum1 : Sum  Inputs=+|+
  Terminator : Terminator
  Terminator1 : Terminator
  alphadot : Outport
  wires:
  Product2/1 -> alphadot/1  "alphadot"
  "[Udot Vdot Wdot]"/1 -> Demux/1
  "[U V W]"/1 -> Demux1/1
  Demux1/2 -> Terminator1/1
  Sum/1 -> Product2/1
  Product/1 -> Sum/2  "U Wdot"
  Product1/1 -> Sum/1  "W Udot"
  Sum1/1 -> Product2/2  "U^2 + W^2"
  Math Function1/1 -> Sum1/2
  Math Function/1 -> Sum1/1
  Demux1/3 -> Math Function1/1, Product1/2
  Demux1/1 -> Math Function/1, Product/2  "U"
  Demux/2 -> Terminator/1
  Demux/3 -> Product/1  "Wdot"
  Demux/1 -> Product1/1  "Udot"

== system aerosonde_dynamics_with_autopilot/ UAV Dynamics/Propulsion System/Piston Engine/Altitude correction for  Power ==
  note: Altitude correction for Power
  T : Inport
  Math Function : Math  Operator=sqrt  SignedPower=on  SaturateOnIntegerOverflow=on
  Product of Elements : Product  Inputs=/
  "Sea-level temperature " : Gain  Gain=TSL  SaturateOnIntegerOverflow=on  OutDataTypeStr=Inherit: Same as input  ParamDataTypeStr=Inherit: Same as input
  Power correction : Outport
  wires:
  T/1 -> Product of Elements/1
  Math Function/1 -> Power correction/1
  "Sea-level temperature "/1 -> Math Function/1
  Product of Elements/1 -> "Sea-level temperature "/1

== system aerosonde_dynamics_with_autopilot/ UAV Dynamics/Propulsion System/Piston Engine/Intake ==
  Thr : Inport  OutDataTypeStr=double  PortDimensions=1
  P_atm : Inport  Port=2  OutDataTypeStr=double  PortDimensions=1
  Get MAP : Product  InputSameDT=on  SaturateOnIntegerOverflow=on  OutDataTypeStr=Inherit: Same as first input
  MAP min : Constant  Value=as.MAPmin
  Saturation : Saturate  UpperLimit=inf  LowerLimit=as.MAPmin
  Sum : Sum  Inputs=|+-  InputSameDT=on  SaturateOnIntegerOverflow=on  OutDataTypeStr=Inherit: Same as first input
  Sum1 : Sum  Inputs=|++  InputSameDT=on  SaturateOnIntegerOverflow=on  OutDataTypeStr=Inherit: Same as first input
  kPa : Gain  Gain=1/1000  SaturateOnIntegerOverflow=on  OutDataTypeStr=Inherit: Same as input  ParamDataTypeStr=Inherit: Same as input
  MAP : Outport
  wires:
  Saturation/1 -> MAP/1
  P_atm/1 -> kPa/1
  Thr/1 -> Get MAP/1
  MAP min/1 -> Sum/2, Sum1/2
  kPa/1 -> Sum/1
  Sum/1 -> Get MAP/2
  Get MAP/1 -> Sum1/1
  Sum1/1 -> Saturation/1

== matlab function aerosonde_dynamics_with_autopilot/AoA Sensor Model/MATLAB Function ==
  data: alpha_fault_free_rad input; y output; bias_fault_active input; alpha_biased_rad input; drift_fault_active input; alpha_drifted_rad input
function y = fcn(alpha_fault_free_rad, ...
                 bias_fault_active, ...
                 alpha_biased_rad,...
                 drift_fault_active,...
                 alpha_drifted_rad)
TRUE = 1;
FALSE = 0;

if((TRUE  == bias_fault_active ) &&...
   (FALSE == drift_fault_active)  )
    y = alpha_biased_rad;

elseif((FALSE == bias_fault_active ) &&...
       (TRUE == drift_fault_active )  )
    y = alpha_drifted_rad;
else
    y = alpha_fault_free_rad;
end

== matlab function aerosonde_dynamics_with_autopilot/Flight Controller/Trajectory tracker/Calculate along and cross track errors ==
  data: Vel_UAV input; Pos_UAV input; Vel_VL input; Pos_VL input; Y output
function Y = track(Vel_UAV,Pos_UAV,Vel_VL,Pos_VL)

xVL = Pos_VL(1);
yVL = Pos_VL(2);
zVL = Pos_VL(3);

xUAV = Pos_UAV(1);
yUAV = Pos_UAV(2);
zUAV = Pos_UAV(3);

ChiVL = atan2(Vel_VL(2),Vel_VL(1));


% Distance between VL and UAV:
d_NED = [xUAV-xVL; yUAV-yVL; zUAV-zVL];

% Relative velocity between VL and UAV:
dV_NED = Vel_UAV - Vel_VL;

% Rotation matrix from NED to unD:
R = [cos(ChiVL) -sin(ChiVL) 0;
     sin(ChiVL)  cos(ChiVL) 0;
            0           0   1];

        
%----------------------------------------

d_unD = (R)\d_NED;
dV_unD = (R)\dV_NED;

ATD = d_unD(1);
OTD = d_unD(2);

dOTD = dV_unD(2);

%----------------------------------------

Y = [OTD; dOTD; ATD];

== matlab function aerosonde_dynamics_with_autopilot/MATLAB Function ==
  data: alpha_measurement_rad input; p_rad_s input; q_rad_s input; r_rad_s input; phi_rad input; theta_rad input; alpha_est_k1_rad input; V_tas_m_s input; beta_rad input; a_x_m_s2 input; a_z_m_s2 input; Ts_s input; P_k1 input; innovation_k1_rad input; alpha_est_rad output; fault_flag output; P_k output; start_flag input; start_flag output; process_variance input; noise_variance input; alpha_dot_rad_s output; time_s input; innovation_rad output; innovation_covariance output
function [alpha_est_rad, fault_flag,P_k,start_flag,alpha_dot_rad_s,innovation_rad, innovation_covariance] =...
                                       Alpha_UKF_Estimator(alpha_measurement_rad,...
                                                           p_rad_s,q_rad_s, r_rad_s,...
                                                           phi_rad, theta_rad, ...
                                                           alpha_est_k1_rad, V_tas_m_s, ...
                                                           beta_rad, ...
                                                           a_x_m_s2,a_z_m_s2, ...
                                                           Ts_s, P_k1, innovation_k1_rad, ...
                                                           start_flag, ...
                                                           process_variance, ...
                                                           noise_variance, ...
                                                           time_s)
    
    TRUE  = 1;
    FALSE = 0;
     
    Q = process_variance^2;
    R = noise_variance^2;  

    H = 1;

    %% Prediction step
    g_m_s2  = 9.80665;
    c_phi   = cos(phi_rad      );
    c_theta = cos(theta_rad    );
    c_alpha = cos(alpha_est_k1_rad);

    s_theta = sin(theta_rad);
    s_alpha = sin(alpha_est_k1_rad);
    c_beta  = cos(beta_rad);

    t_beta  = tan(beta_rad);

    alpha_dot_rad_s = q_rad_s + ...
                     (g_m_s2*c_phi*c_theta*c_alpha + g_m_s2*s_theta*s_alpha - ...
                      a_x_m_s2*s_alpha + a_z_m_s2*c_alpha) / (V_tas_m_s * c_beta) - ...
                      (p_rad_s * c_alpha + r_rad_s * s_alpha) * t_beta;

    alpha_pred_rad = alpha_est_k1_rad + alpha_dot_rad_s * Ts_s;

    % Sytem Jacobian
    F =  (g_m_s2*c_phi*c_theta*-1*s_alpha + g_m_s2*s_theta*c_alpha - ...
          -1* a_x_m_s2*c_alpha - a_z_m_s2*s_alpha) / (V_tas_m_s * c_beta) - ...
          (r_rad_s * c_alpha - p_rad_s * s_alpha) * t_beta;
    
    F = (1+Ts_s*F);

    % Error Covariance Matrix
    P_k = F * P_k1 * F' + Q;

    innovation_rad = (alpha_measurement_rad - alpha_pred_rad);

    % Kalman Gain
    K = P_k*H'/(H*P_k*H' + R);


    %% Update Step
    alpha_est_rad = alpha_pred_rad + K*innovation_rad;
    innovation_covariance = (H*P_k*H' + R);

    P_k = (1 - K*H)* P_k;

    %% Residual
    epsilon_rad = deg2rad(2);
    if (abs(innovation_rad) > epsilon_rad )
        fault_flag = TRUE;
    else
        fault_flag = FALSE;
    end



end
